simulink model "EMF"  (R2023a)
settings: Solver=VariableStepAuto  StartTime=0.0  StopTime=10.0  RelTol=1e-3
undefined symbols (not defined in the file or in its folder): Il, Kb, Kt, L, R
settings Model: Creator=paragmraw  LastModifiedBy=paragmraw

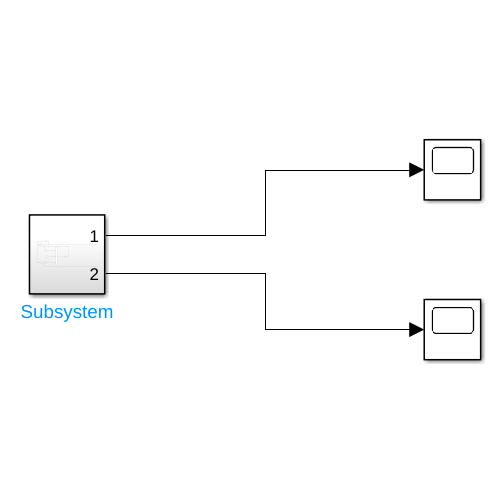
[thumbnail: Simulink's stored preview of the top-level diagram]
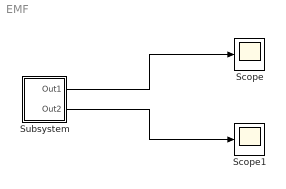
== system EMF ==
  Scope : Scope
  Scope1 : Scope
  Subsystem : Subsystem
  wires:
  Subsystem/1(Out1) -> Scope/1
  Subsystem/2(Out2) -> Scope1/1

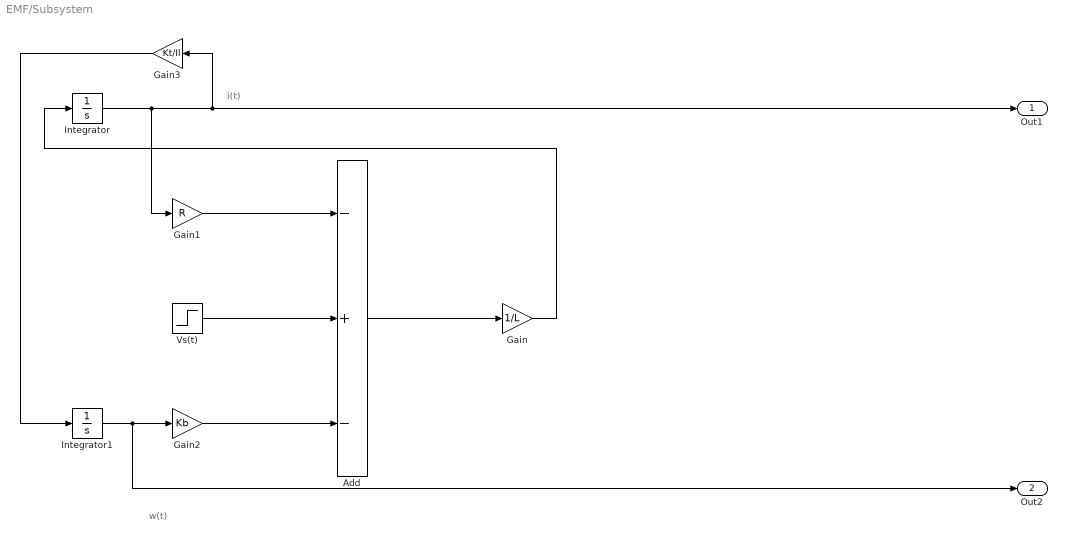
== system EMF/Subsystem ==
  note: w(t)
  note: i(t)
  Add : Sum  Inputs=-+-
  Gain : Gain  Gain=1/L
  Gain1 : Gain  Gain=R
  Gain2 : Gain  Gain=Kb
  Gain3 : Gain  Gain=Kt/Il
  Integrator : Integrator
  Integrator1 : Integrator
  Vs(t) : Step  SampleTime=0
  Out1 : Outport
  Out2 : Outport  Port=2
  wires:
  Add/1 -> Gain/1
  Integrator/1 -> Gain1/1, Out1/1, Gain3/1
  Gain2/1 -> Add/3
  Vs(t)/1 -> Add/2
  Gain1/1 -> Add/1
  Gain3/1 -> Integrator1/1
  Gain/1 -> Integrator/1
  Integrator1/1 -> Out2/1, Gain2/1
